simulink model "model"  (R2019b)
settings: Solver=VariableStepAuto  StartTime=0.0  StopTime=500  RelTol=1e-3
undefined symbols (not defined in the file): Duration, Effort, JointName, StartTime
libraries: robotlib x10, simulink x4
settings Model: Creator=AngelofDeath  LastModifiedBy=AngelofDeath

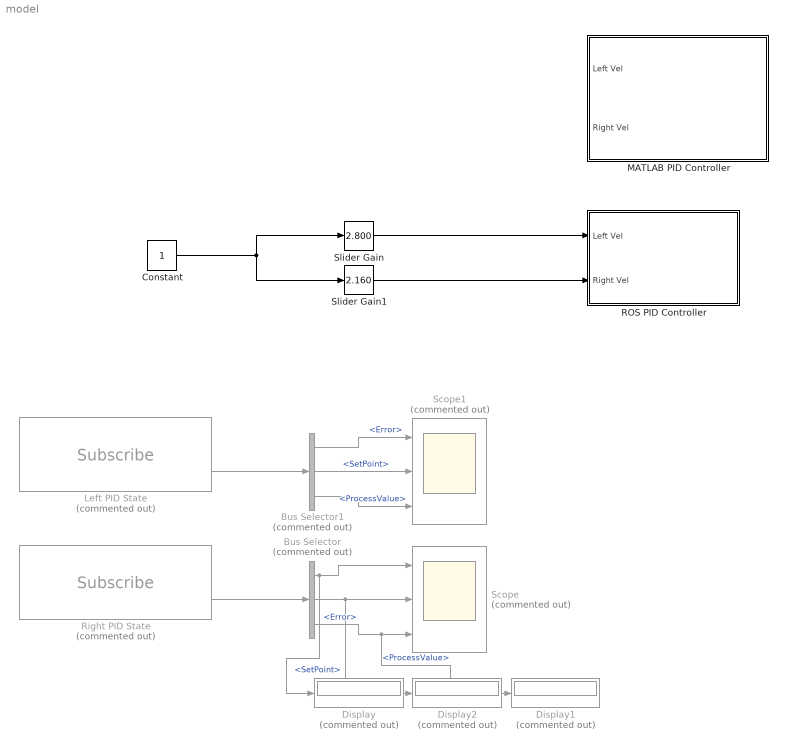
== system model ==
  Bus Selector : BusSelector  Commented=on  OutputSignals=Error,SetPoint,ProcessValue
  Bus Selector1 : BusSelector  Commented=on  OutputSignals=Error,SetPoint,ProcessValue
  Constant : Constant
  Display : Display  Commented=on
      settings: Decimation=3
  Display1 : Display  Commented=on
      settings: Decimation=3
  Display2 : Display  Commented=on
      settings: Decimation=3
  Left PID State : robotlib/Subscribe  Commented=on  topicSource=Select from ROS network  topic=/joint_left_velocity_controller/state  messageType=control_msgs/JointControllerState  sampleTime=-1  messageQueueLength=1
      settings: SourceProductName=ROS Toolbox
  MATLAB PID Controller : Subsystem
  ROS PID Controller : Subsystem
  Right PID State : robotlib/Subscribe  Commented=on  topicSource=Select from ROS network  topic=/joint_right_velocity_controller/state  messageType=control_msgs/JointControllerState  sampleTime=-1  messageQueueLength=1
      settings: SourceProductName=ROS Toolbox
  Scope : Scope  Commented=on  NumInputPorts=3
  Scope1 : Scope  Commented=on  NumInputPorts=3
  Slider Gain : simulink/Math Operations/Slider Gain  gain=2.800  low=-4  high=4
  Slider Gain1 : simulink/Math Operations/Slider Gain  gain=2.160  low=-4  high=4
  wires:
  Constant/1 -> Slider Gain1/1, Slider Gain/1
  Right PID State/2 -> Bus Selector/1
  Bus Selector/2 -> Display2/1, Scope/2  "<SetPoint>"
  Bus Selector/1 -> Display/1, Scope/1  "<Error>"
  Bus Selector/3 -> Display1/1, Scope/3  "<ProcessValue>"
  Bus Selector1/3 -> Scope1/3  "<ProcessValue>"
  Bus Selector1/1 -> Scope1/1  "<Error>"
  Bus Selector1/2 -> Scope1/2  "<SetPoint>"
  Left PID State/2 -> Bus Selector1/1
  Slider Gain/1 -> ROS PID Controller/1(Left Vel)
  Slider Gain1/1 -> ROS PID Controller/2(Right Vel)

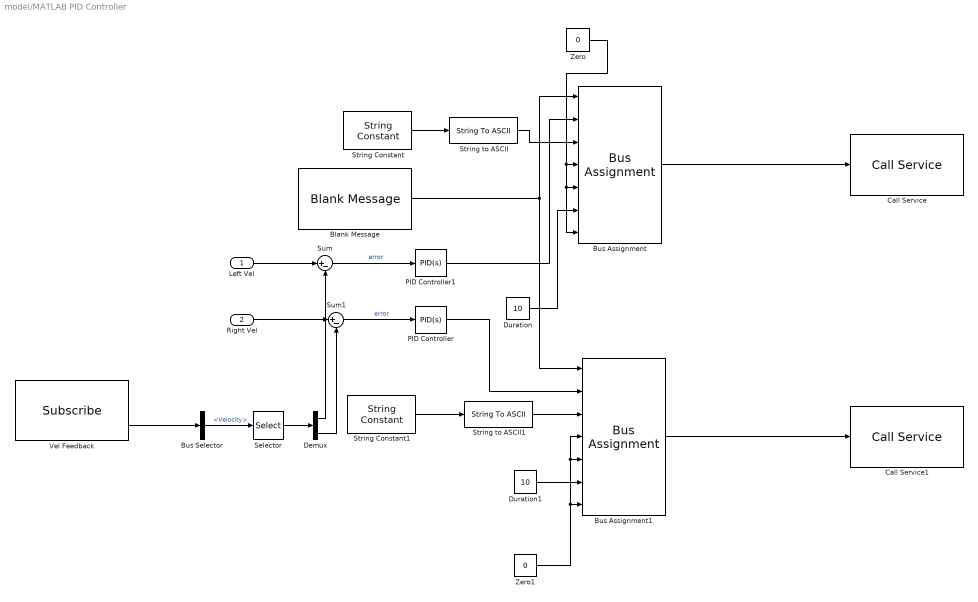
== system model/MATLAB PID Controller ==
  Left Vel : Inport
  Right Vel : Inport  Port=2
  Blank Message : robotlib/Blank Message  messageClass=Service Request  entityType=gazebo_msgs/ApplyJointEffort  messageType=gazebo_msgs/ApplyJointEffortRequest  SampleTime=inf
      settings: SourceProductName=ROS Toolbox
  Bus Assignment : BusAssignment  AssignedSignals=Effort,JointName,StartTime.Sec,StartTime.Nsec,Duration.Sec,Duration.Nsec
  Bus Assignment1 : BusAssignment  AssignedSignals=Effort,JointName,StartTime.Sec,StartTime.Nsec,Duration.Sec,Duration.Nsec
  Bus Selector : BusSelector  OutputSignals=Velocity
  Call Service : robotlib/Call Service  topicSource=Select from ROS network  service=/gazebo/apply_joint_effort  serviceType=gazebo_msgs/ApplyJointEffort  connectionTimeout=5  keepPersistent=off  ShowErrorCodeOutput=on
      settings: SourceProductName=ROS Toolbox  SourceProductBaseCode=RR
  Call Service1 : robotlib/Call Service  topicSource=Select from ROS network  service=/gazebo/apply_joint_effort  serviceType=gazebo_msgs/ApplyJointEffort  connectionTimeout=5  keepPersistent=off  ShowErrorCodeOutput=on
      settings: SourceProductName=ROS Toolbox  SourceProductBaseCode=RR
  Demux : Demux  Outputs=2
  Duration : Constant  Value=10
  Duration1 : Constant  Value=10
  PID Controller : simulink/Continuous/PID Controller  Controller=PID  Form=Parallel  TimeDomain=Continuous-time  SampleTime=-1  IntegratorMethod=Forward Euler  FilterMethod=Forward Euler  ControllerParametersSource=internal  P=0.08  I=0.02  D=0  UseFilter=on  N=100  TunerSelectOption=Transfer Function Based (PID Tuner App)  InitialConditionSource=internal  InitialConditionForIntegrator=0  InitialConditionForFilter=0  DifferentiatorICPrevScaledInput=0  ExternalReset=none  TrackingMode=off  Kt=1  LimitOutput=off  UpperSaturationLimit=inf  LowerSaturationLimit=-inf  LinearizeAsGain=on  AntiWindupMode=none  Kb=1  POutMin=[]  POutMax=[]  IOutMin=[]  IOutMax=[]  DOutMin=[]  DOutMax=[]  NOutMin=[]  NOutMax=[]  SumOutMin=[]  SumOutMax=[]  SaturationOutMin=[]  SaturationOutMax=[]  PParamMin=[]  PParamMax=[]  IParamMin=[]  IParamMax=[]  DParamMin=[]  DParamMax=[]  NParamMin=[]  NParamMax=[]  KbParamMin=[]  KbParamMax=[]  KtParamMin=[]  KtParamMax=[]  KbOutMin=[]  KbOutMax=[]  KtOutMin=[]  KtOutMax=[]  IntegratorOutMin=[]  IntegratorOutMax=[]  FilterOutMin=[]  FilterOutMax=[]  SumI1OutMin=[]  SumI1OutMax=[]  SumI2OutMin=[]  SumI2OutMax=[]  SumI3OutMin=[]  SumI3OutMax=[]  SumI4OutMin=[]  SumI4OutMax=[]  SumDOutMin=[]  SumDOutMax=[]  DifferentiatorOutMin=[]  DifferentiatorOutMax=[]  FilterDiffOutCoefMin=[]  FilterDiffOutCoefMax=[]  ReciprocalOutMin=[]  ReciprocalOutMax=[]  SumDenOutMin=[]  SumDenOutMax=[]  SumNumOutMin=[]  SumNumOutMax=[]  DivideOutMin=[]  DivideOutMax=[]  IntegratorContinuousStateAttributes=''  IntegratorStateMustResolveToSignalObject=off  IntegratorRTWStateStorageClass=Auto  FilterContinuousStateAttributes=''  FilterStateMustResolveToSignalObject=off  FilterRTWStateStorageClass=Auto  ParallelPVariant=InternalParameters  IdealPVariant=Disabled  IVariant=InternalParameters  DVariant=InternalParameters  IntegratorVariant=Continuous  SatVariant=Disabled  AWVariant=Passthrough  PCopyVariant=Disabled  TRVariant=Disabled  FdbkBlocksVariant=Forward  IdealPFdbkVariant=Disabled  SatFdbkVariant=Disabled  DerivativeFilterVariant=ContFilter  NVariant=InternalParameters  NCopyVariant=Disabled  FilterICVariant=InternalICsFilter  IntegratorICVariant=InternalICs  ExternalResetVariant=Disabled  TRSumVariant=Passthrough  SumFdbkVariant=Disabled  SumVariant=Sum_PID
  PID Controller1 : simulink/Continuous/PID Controller  Controller=PID  Form=Parallel  TimeDomain=Continuous-time  SampleTime=-1  IntegratorMethod=Forward Euler  FilterMethod=Forward Euler  ControllerParametersSource=internal  P=0.08  I=0.02  D=0  UseFilter=on  N=100  TunerSelectOption=Transfer Function Based (PID Tuner App)  InitialConditionSource=internal  InitialConditionForIntegrator=0  InitialConditionForFilter=0  DifferentiatorICPrevScaledInput=0  ExternalReset=none  TrackingMode=off  Kt=1  LimitOutput=off  UpperSaturationLimit=inf  LowerSaturationLimit=-inf  LinearizeAsGain=on  AntiWindupMode=none  Kb=1  POutMin=[]  POutMax=[]  IOutMin=[]  IOutMax=[]  DOutMin=[]  DOutMax=[]  NOutMin=[]  NOutMax=[]  SumOutMin=[]  SumOutMax=[]  SaturationOutMin=[]  SaturationOutMax=[]  PParamMin=[]  PParamMax=[]  IParamMin=[]  IParamMax=[]  DParamMin=[]  DParamMax=[]  NParamMin=[]  NParamMax=[]  KbParamMin=[]  KbParamMax=[]  KtParamMin=[]  KtParamMax=[]  KbOutMin=[]  KbOutMax=[]  KtOutMin=[]  KtOutMax=[]  IntegratorOutMin=[]  IntegratorOutMax=[]  FilterOutMin=[]  FilterOutMax=[]  SumI1OutMin=[]  SumI1OutMax=[]  SumI2OutMin=[]  SumI2OutMax=[]  SumI3OutMin=[]  SumI3OutMax=[]  SumI4OutMin=[]  SumI4OutMax=[]  SumDOutMin=[]  SumDOutMax=[]  DifferentiatorOutMin=[]  DifferentiatorOutMax=[]  FilterDiffOutCoefMin=[]  FilterDiffOutCoefMax=[]  ReciprocalOutMin=[]  ReciprocalOutMax=[]  SumDenOutMin=[]  SumDenOutMax=[]  SumNumOutMin=[]  SumNumOutMax=[]  DivideOutMin=[]  DivideOutMax=[]  IntegratorContinuousStateAttributes=''  IntegratorStateMustResolveToSignalObject=off  IntegratorRTWStateStorageClass=Auto  FilterContinuousStateAttributes=''  FilterStateMustResolveToSignalObject=off  FilterRTWStateStorageClass=Auto  ParallelPVariant=InternalParameters  IdealPVariant=Disabled  IVariant=InternalParameters  DVariant=InternalParameters  IntegratorVariant=Continuous  SatVariant=Disabled  AWVariant=Passthrough  PCopyVariant=Disabled  TRVariant=Disabled  FdbkBlocksVariant=Forward  IdealPFdbkVariant=Disabled  SatFdbkVariant=Disabled  DerivativeFilterVariant=ContFilter  NVariant=InternalParameters  NCopyVariant=Disabled  FilterICVariant=InternalICsFilter  IntegratorICVariant=InternalICs  ExternalResetVariant=Disabled  TRSumVariant=Passthrough  SumFdbkVariant=Disabled  SumVariant=Sum_PID
  Selector : Selector  IndexOptions=Index vector (dialog)  Indices=[1 2]  OutputSizes=1
  String Constant : StringConstant  String='wheel_left_joint'
  String Constant1 : StringConstant  String="\"wheel_right_joint\""
  String to ASCII : StringToASCII  OutputVectorSize=128
  String to ASCII1 : StringToASCII  OutputVectorSize=128
  Sum : Sum  Inputs=|+-
  Sum1 : Sum  Inputs=|+-
  Vel Feedback : robotlib/Subscribe  topicSource=Select from ROS network  topic=/joint_states  messageType=sensor_msgs/JointState  sampleTime=-1  messageQueueLength=1
      settings: SourceProductName=ROS Toolbox
  Zero : Constant  Value=0
  Zero1 : Constant  Value=0
  wires:
  Vel Feedback/2 -> Bus Selector/1
  Demux/1 -> Sum/2
  Sum/1 -> PID Controller1/1  "error"
  Left Vel/1 -> Sum/1
  Right Vel/1 -> Sum1/1
  Demux/2 -> Sum1/2
  Sum1/1 -> PID Controller/1  "error"
  Blank Message/1 -> Bus Assignment/1, Bus Assignment1/1
  Zero/1 -> Bus Assignment/7, Bus Assignment/5, Bus Assignment/4
  Duration/1 -> Bus Assignment/6
  PID Controller1/1 -> Bus Assignment/2
  PID Controller/1 -> Bus Assignment1/2
  Bus Assignment/1 -> Call Service/1
  Duration1/1 -> Bus Assignment1/6
  Zero1/1 -> Bus Assignment1/4, Bus Assignment1/5, Bus Assignment1/7
  Bus Assignment1/1 -> Call Service1/1
  Bus Selector/1 -> Selector/1  "<Velocity>"
  Selector/1 -> Demux/1
  String Constant/1 -> String to ASCII/1
  String to ASCII/1 -> Bus Assignment/3
  String to ASCII1/1 -> Bus Assignment1/3
  String Constant1/1 -> String to ASCII1/1

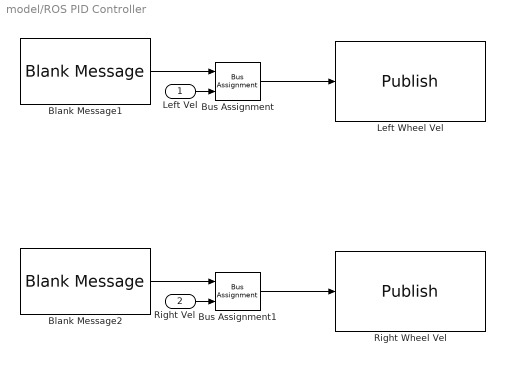
== system model/ROS PID Controller ==
  Left Vel : Inport
  Right Vel : Inport  Port=2
  Blank Message1 : robotlib/Blank Message  messageClass=Message  entityType=std_msgs/Float64  messageType=std_msgs/Float64  SampleTime=0.01
      settings: SourceProductName=ROS Toolbox
  Blank Message2 : robotlib/Blank Message  messageClass=Message  entityType=std_msgs/Float64  messageType=std_msgs/Float64  SampleTime=0.01
      settings: SourceProductName=ROS Toolbox
  Bus Assignment : BusAssignment  DialogController=Simulink.DDGSource_BusAssignment  AssignedSignals=Data
  Bus Assignment1 : BusAssignment  DialogController=Simulink.DDGSource_BusAssignment  AssignedSignals=Data
  Left Wheel Vel : robotlib/Publish  topicSource=Select from ROS network  topic=/joint_left_velocity_controller/command  messageType=std_msgs/Float64  messageQueueLength=1
      settings: SourceProductName=ROS Toolbox
  Right Wheel Vel : robotlib/Publish  topicSource=Select from ROS network  topic=/joint_right_velocity_controller/command  messageType=std_msgs/Float64  messageQueueLength=1
      settings: SourceProductName=ROS Toolbox
  wires:
  Blank Message2/1 -> Bus Assignment1/1
  Bus Assignment/1 -> Left Wheel Vel/1
  Blank Message1/1 -> Bus Assignment/1
  Bus Assignment1/1 -> Right Wheel Vel/1
  Left Vel/1 -> Bus Assignment/2
  Right Vel/1 -> Bus Assignment1/2
